simulink library "WaitResponse"  (R2015a)
settings: Solver=ode45  StartTime=0.0  StopTime=10.0  RelTol=1e-3
values from neighbouring files (symbols this model uses):
  LEVEL0 = uint8(0)    [const.m]
  LEVEL1 = uint8(1)    [const.m]
  LEVEL2 = uint8(2)    [const.m]
settings Model: Creator=mbd_user  LastModifiedBy=mbd_user

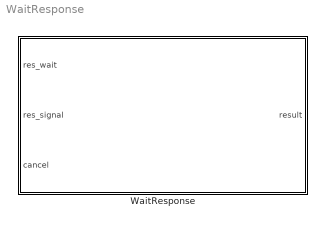
== system WaitResponse ==
  WaitResponse : Subsystem  TreatAsAtomicUnit=on

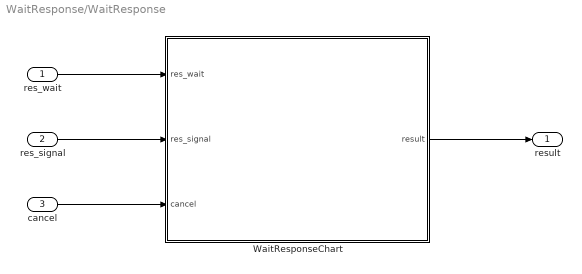
== system WaitResponse/WaitResponse ==
  res_wait : Inport
  res_signal : Inport  Port=2
  cancel : Inport  Port=3
  WaitResponseChart : Stateflow chart  TreatAsAtomicUnit=on
  result : Outport
  wires:
  res_wait/1 -> WaitResponseChart/1(res_wait)
  res_signal/1 -> WaitResponseChart/2(res_signal)
  cancel/1 -> WaitResponseChart/3(cancel)
  WaitResponseChart/1(result) -> result/1

== stateflow chart WaitResponse/WaitResponseChart ==
  state STOP
    en :
    result = LEVEL0;
  state WAIT
    en :
    result = LEVEL1;
  state SUCCESS
    en :
    result = LEVEL2;
  (default) -> STOP
  STOP -> WAIT : [res_wait == ON]
  WAIT -> STOP [order 1] : [cancel == ON || after(100,msec)]
  WAIT -> SUCCESS [order 2] : [res_signal == ON]
  SUCCESS -> STOP
  data: res_wait input; res_signal input; cancel input; result output =OFF; OFF parameter; ON parameter; LEVEL0 parameter; LEVEL1 parameter; LEVEL2 parameter
